simulink model "H2_z"  (R2020b)
settings: Solver=VariableStepAuto  StartTime=0.0  StopTime=10.0  RelTol=1e-3
settings Model: Creator=user  LastModifiedBy=user
settings DataIOCC: SaveOutput=off  SaveTime=off

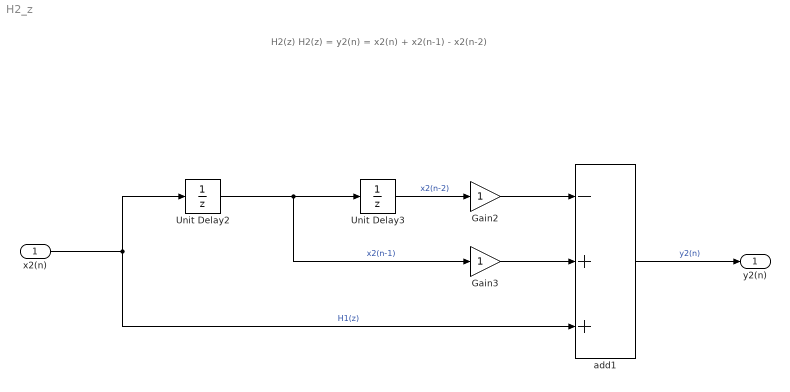
== system H2_z ==
  note: H2(z)
      |
      | H2(z) = y2(n) = x2(n) + x2(n-1) - x2(n-2)
  x2(n) : Inport  OutDataTypeStr=double  PortDimensions=1  SampleTime=0
  Gain2 : Gain
  Gain3 : Gain
  Unit Delay2 : UnitDelay  SampleTime=-1  HasFrameUpgradeWarning=on
  Unit Delay3 : UnitDelay  SampleTime=-1  HasFrameUpgradeWarning=on
  add1 : Sum  Inputs=-++
  y2(n) : Outport  OutDataTypeStr=double  PortDimensions=1  SampleTime=0
  wires:
  x2(n)/1 -> add1/3, Unit Delay2/1  "H1(z)"
  add1/1 -> y2(n)/1  "y2(n)"
  Gain2/1 -> add1/1
  Unit Delay3/1 -> Gain2/1  "x2(n-2)"
  Unit Delay2/1 -> Unit Delay3/1, Gain3/1  "x2(n-1)"
  Gain3/1 -> add1/2
